simulink model "P4_Modelo_4_11_RealimEstim_ContrInt"  (R2025b)
settings: Solver=VariableStepAuto  StartTime=0.0  StopTime=10.0  RelTol=1e-3
undefined symbols (not defined in the file): A, B, C, K, k_e, L, p
settings Model: Creator=Pc24
settings DebuggingCC: UnconnectedInputMsg=warning  UnconnectedOutputMsg=warning  UnconnectedLineMsg=warning
settings ModelReferenceCC: EnableRefExpFcnMdlSchedulingChecks=on
settings RTWCC: GPUComputeCapability=3.5  DLArmComputeVersion=19.05

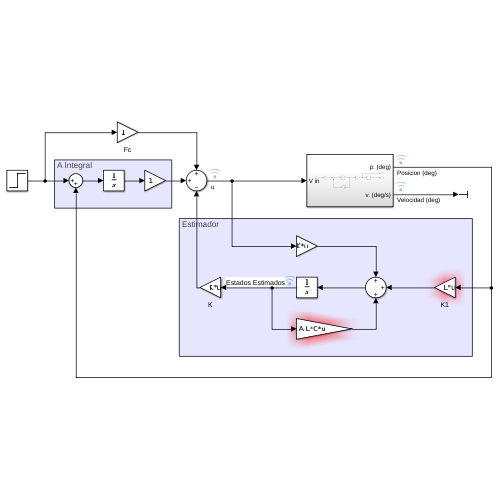
[thumbnail: Simulink's stored preview of the top-level diagram]
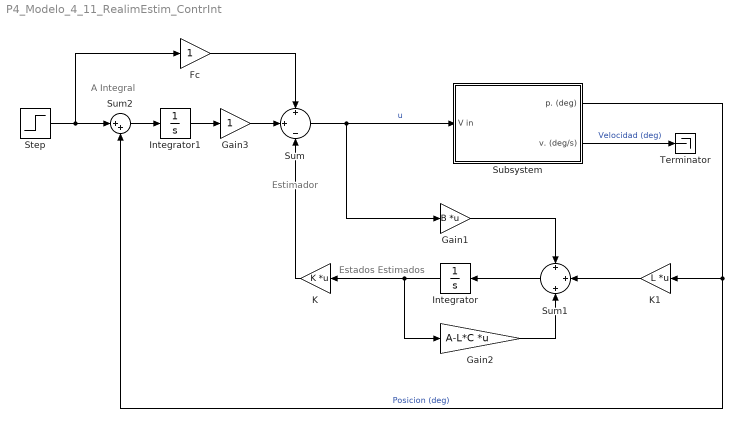
== system P4_Modelo_4_11_RealimEstim_ContrInt ==
  note: A Integral
  note: Estimador
  note: Estados Estimados
  Fc : Gain
  Gain1 : Gain  Gain=B  Multiplication=Matrix(K*u)
  Gain2 : Gain  Gain=A-L*C  Multiplication=Matrix(K*u)
  Gain3 : Gain
  Integrator : Integrator
  Integrator1 : Integrator
  K : Gain  Gain=K  Multiplication=Matrix(K*u)
  K1 : Gain  Gain=L  Multiplication=Matrix(K*u)
  Step : Step  SampleTime=0
  Subsystem : Subsystem
  Sum : Sum  Inputs=+|+|-
  Sum1 : Sum  Inputs=+|+|+
  Sum2 : Sum  Inputs=|++
  Terminator : Terminator
  wires:
  Sum/1 -> Gain1/1, Subsystem/1(V in)  "u"
  Subsystem/2(v. (deg/s)) -> Terminator/1  "Velocidad (deg)"
  Subsystem/1(p. (deg)) -> K1/1, Sum2/2  "Posicion (deg)"
  Step/1 -> Sum2/1, Fc/1
  Fc/1 -> Sum/1
  K1/1 -> Sum1/2
  Gain1/1 -> Sum1/1
  Sum1/1 -> Integrator/1
  Integrator/1 -> Gain2/1, K/1
  Gain2/1 -> Sum1/3
  Integrator1/1 -> Gain3/1
  Sum2/1 -> Integrator1/1
  Gain3/1 -> Sum/2
  K/1 -> Sum/3

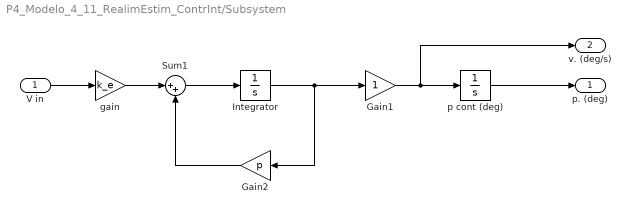
== system P4_Modelo_4_11_RealimEstim_ContrInt/Subsystem ==
  V in : Inport
  Gain1 : Gain
  Gain2 : Gain  Gain=p
  Integrator : Integrator
  Sum1 : Sum  Inputs=|++
  gain : Gain  Gain=k_e
  p cont (deg) : Integrator
  p. (deg) : Outport
  v. (deg/s) : Outport  Port=2
  wires:
  V in/1 -> gain/1
  p cont (deg)/1 -> p. (deg)/1
  Integrator/1 -> Gain2/1, Gain1/1
  Gain2/1 -> Sum1/2
  Gain1/1 -> v. (deg/s)/1, p cont (deg)/1
  Sum1/1 -> Integrator/1
  gain/1 -> Sum1/1
